simulink model "sampleModel1819"  (R2023a)
settings: Solver=VariableStepAuto  StartTime=0.0  StopTime=10.0  RelTol=1e-3
libraries: hdlsllib x4, simulink x2
settings Model: Creator=user1  LastModifiedBy=user1

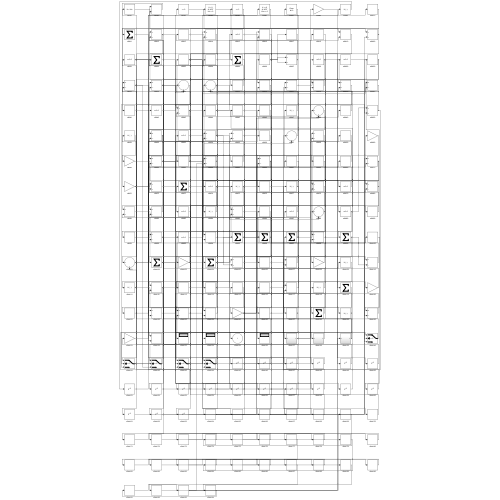
[thumbnail: Simulink's stored preview of the top-level diagram]
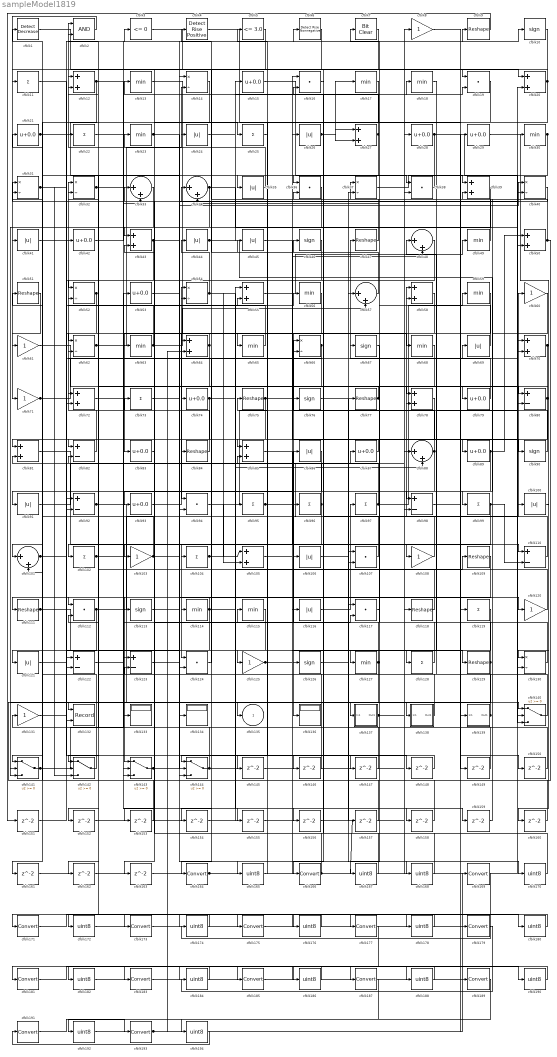
== system sampleModel1819 ==
  cfblk1 : simulink/Logic and Bit Operations/Detect Decrease  vinit=0.0  OutDataTypeStr=boolean
      settings: LibrarySourceBlock=|
      | hdlsllib/Logic and Bit
      | Operations/Detect
      | Decrease
  cfblk{10,46,67,76,90,113,126} (7 alike) : Signum
  cfblk{24,26,35,41,44..45,69,86,91,100,106,116,121} (13 alike) : Abs  SaturateOnIntegerOverflow=off
  cfblk{33..34,48,57,88,101} (6 alike) : Sum  Inputs=|++
  cfblk{11,22,25,73,95..97,99,102,104,119,128} (12 alike) : Sum  Inputs=+
  cfblk{8,60..61,71,103,108,120,125,131} (9 alike) : Gain
  cfblk{12,20,27,39,43,50,55,58,64,70,72,78,81,85,105} (15 alike) : Sum
  cfblk{16,19,36,38,94,107,112,117,124} (9 alike) : DotProduct  OutDataTypeStr=Inherit: Inherit via internal rule
  cfblk{9,47,51,75,77,84,109,111,118,129} (10 alike) : Reshape
  cfblk{80,82,92,98,110,122..123} (7 alike) : Sum  Inputs=+-
  cfblk{13,17..18,23,30,49,56,59,63,65,68,114..115,127} (14 alike) : MinMax
  cfblk{14,31..32,37,40,52,54,62,66,130} (10 alike) : Product  Inputs=*/  RndMeth=Zero  SaturateOnIntegerOverflow=on
  cfblk132 : Record  FileSettingsInternal="{\"entries\":[{\"content\":{\"excelSettings\":{\"content\":{},\"type\":\"Streamout.ExcelSettings\"}},\"type\":\"Streamout.FileSettingStorage\",\"uuid\":\"\"}],\"packageUris\":[\"http:\\/\\/schema.mathworks.com\\/mf0\\/streamout_blocks\\/R2020a\"],\"version\":\"1.0\"}"  Layout=[1 1]  SignalsInternal="{\"entries\":[{\"content\":{\"signals\":[{\"content\":{\"blockPath\":[],\"dimensions\":[1],\"domain\":\"\",\"lineColor\":\"#a2142f\",\"plots\":[1],\"port\":1,\"signalID\":4319,\"signalName\":\"XY Graph:1\"},\"type\":\"RecordBlkView.Signal\",\"uuid\":\"\"},{\"content\":{\"blockPath\":[],\"dimensions\":[1],\"domain\":\"\",\"lineColor\":\"#139fff\",\"plots\":[1],\"port\":2,\"signalID\":4322,\"signalName\":\"XY Graph:2\"},\"type\":\"RecordBlkView.Signal\",\"uuid\":\"\"}]},\"type\":\"RecordBlkView.InputSignals\",\"uuid\":\"\"}],\"packageUris\":[\"http:\\/\\/schema.mathworks.com\\/mf0\\/streamout_blocks\\/R2020a\"],\"version\":\"1.0\"}"  VisualizationBindings="{\"xyplotplugin\":{\"info\":[{\"series\":[{\"bindingParametersList\":[{\"parameter\":\"X-Axis\",\"signalID\":4319,\"signalName\":\"XY Graph:1\"},{\"parameter\":\"Y-Axis\",\"signalID\":4322,\"signalName\":\"XY Graph:2\"}],\"seriesID\":21637}],\"subplotID\":1}]}}"  CompatibilityTag=XY  st=-1
  cfblk133 : Display
  cfblk134 : Display
  cfblk136 : Display
  cfblk137 : Subsystem
      settings: LibrarySourceBlock=|
      | hdlsllib/Ports &
      | Subsystems/Subsystem
  cfblk138 : Subsystem
      settings: LibrarySourceBlock=|
      | hdlsllib/Ports &
      | Subsystems/Subsystem
  cfblk139 : Subsystem
      settings: LibrarySourceBlock=|
      | hdlsllib/Ports &
      | Subsystems/Subsystem
  cfblk{140..144} (5 alike) : Switch  SaturateOnIntegerOverflow=off  InputSameDT=off
  cfblk{145..163} (19 alike) : Delay  SampleTime=1
  cfblk{15,21,28..29,42,53,74,79,83,87,89,93} (12 alike) : Bias  Bias=0.0  SaturateOnIntegerOverflow=off
  cfblk{164,166,169,171,173,175,177,179,181,183,185,187,189,191,193} (15 alike) : DataTypeConversion  SaturateOnIntegerOverflow=off  RndMeth=Floor
  cfblk{165,167..168,170,172,174,176,178,180,182,184,186,188,190,192,194} (16 alike) : DataTypeConversion  OutDataTypeStr=uint8  SaturateOnIntegerOverflow=off  RndMeth=Floor
  cfblk2 : Logic  AllPortsSameDT=off  OutDataTypeStr=boolean
  cfblk3 : hdlsllib/Logic and Bit Operations/Compare To Zero  relop=<=  OutDataTypeStr=boolean
  cfblk4 : hdlsllib/Logic and Bit Operations/Detect Rise Positive  vinit=0  OutDataTypeStr=boolean
  cfblk5 : hdlsllib/Logic and Bit Operations/Compare To Constant  relop=<=  const=3.0  OutDataTypeStr=boolean
  cfblk6 : hdlsllib/Logic and Bit Operations/Detect Rise Nonnegative  vinit=0  OutDataTypeStr=boolean
  cfblk7 : simulink/Logic and Bit Operations/Bit Clear  iBit=0
      settings: LibrarySourceBlock=|
      | hdlsllib/Logic and Bit
      | Operations/Bit Clear
  cfblk135 : Outport  VectorParamsAs1DForOutWhenUnconnected=off
  wires:
  cfblk56/1 -> cfblk83/1
  cfblk13/1 -> cfblk65/1
  cfblk89/1 -> cfblk50/1, cfblk154/1
  cfblk1/1 -> cfblk20/1
  cfblk119/1 -> cfblk125/1
  cfblk54/1 -> cfblk44/1, cfblk105/2, cfblk156/1
  cfblk44/1 -> cfblk99/1, cfblk18/1
  cfblk95/1 -> cfblk60/1, cfblk80/2
  cfblk79/1 -> cfblk47/1
  cfblk49/1 -> cfblk23/1
  cfblk97/1 -> cfblk59/1, cfblk51/1
  cfblk144/1 -> cfblk131/1, cfblk98/2
  cfblk29/1 -> cfblk130/1
  cfblk108/1 -> cfblk58/1
  cfblk138/1(Out1) -> cfblk73/1
  cfblk59/1 -> cfblk136/1
  cfblk143/1 -> cfblk14/1, cfblk40/2
  cfblk96/1 -> cfblk102/1, cfblk82/2
  cfblk55/1 -> cfblk49/1
  cfblk93/1 -> cfblk54/1
  cfblk21/1 -> cfblk25/1, cfblk144/3, cfblk146/1
  cfblk92/1 -> cfblk137/1(In1), cfblk112/1
  cfblk130/1 -> cfblk86/1
  cfblk43/1 -> cfblk40/1, cfblk72/2
  cfblk50/1 -> cfblk132/1, cfblk24/1
  cfblk2/1 -> cfblk71/1
  cfblk19/1 -> cfblk98/1
  cfblk112/1 -> cfblk100/1, cfblk161/1
  cfblk128/1 -> cfblk7/1
  cfblk26/1 -> cfblk17/1, cfblk27/1, cfblk27/2
  cfblk127/1 -> cfblk33/1, cfblk163/1
  cfblk82/1 -> cfblk32/1
  cfblk23/1 -> cfblk134/1, cfblk76/1, cfblk96/1
  cfblk4/1 -> cfblk119/1
  cfblk7/1 -> cfblk106/1
  cfblk109/1 -> cfblk143/1
  cfblk91/1 -> cfblk87/1
  cfblk57/1 -> cfblk34/1
  cfblk10/1 -> cfblk41/1
  cfblk131/1 -> cfblk56/1
  cfblk14/1 -> cfblk123/1
  cfblk3/1 -> cfblk19/1
  cfblk20/1 -> cfblk35/1, cfblk11/1
  cfblk64/1 -> cfblk62/1, cfblk152/1
  cfblk38/1 -> cfblk36/1
  cfblk129/1 -> cfblk75/1, cfblk141/3
  cfblk99/1 -> cfblk124/1, cfblk110/2
  cfblk5/1 -> cfblk164/1
  cfblk103/1 -> cfblk31/1, cfblk165/1
  cfblk71/1 -> cfblk28/1, cfblk54/2
  cfblk126/1 -> cfblk77/1
  cfblk37/1 -> cfblk39/1
  cfblk62/1 -> cfblk14/2, cfblk94/2, cfblk148/1
  cfblk81/1 -> cfblk130/2
  cfblk61/1 -> cfblk79/1
  cfblk63/1 -> cfblk57/2, cfblk22/1, cfblk168/1
  cfblk116/1 -> cfblk97/1
  cfblk70/1 -> cfblk126/1, cfblk144/2
  cfblk90/1 -> cfblk48/1
  cfblk75/1 -> cfblk141/1, cfblk67/1
  cfblk40/1 -> cfblk31/2
  cfblk17/1 -> cfblk43/1
  cfblk125/1 -> cfblk48/2, cfblk129/1, cfblk78/2
  cfblk36/1 -> cfblk114/1
  cfblk30/1 -> cfblk128/1, cfblk133/1
  cfblk102/1 -> cfblk158/1, cfblk159/1
  cfblk80/1 -> cfblk93/1, cfblk78/1
  cfblk15/1 -> cfblk38/1
  cfblk85/1 -> cfblk107/2
  cfblk76/1 -> cfblk138/1(In1)
  cfblk69/1 -> cfblk34/2
  cfblk120/1 -> cfblk45/1
  cfblk72/1 -> cfblk55/2
  cfblk6/1 -> cfblk63/1
  cfblk33/1 -> cfblk141/2
  cfblk27/1 -> cfblk4/1, cfblk121/1
  cfblk46/1 -> cfblk122/2
  cfblk83/1 -> cfblk113/1
  cfblk68/1 -> cfblk94/1
  cfblk58/1 -> cfblk84/1
  cfblk51/1 -> cfblk61/1
  cfblk122/1 -> cfblk117/2
  cfblk18/1 -> cfblk108/1
  cfblk110/1 -> cfblk36/2
  cfblk113/1 -> cfblk66/1
  cfblk74/1 -> cfblk80/1, cfblk88/2, cfblk162/1
  cfblk52/1 -> cfblk132/2, cfblk92/2
  cfblk11/1 -> cfblk42/1
  cfblk124/1 -> cfblk64/1
  cfblk107/1 -> cfblk46/1
  cfblk35/1 -> cfblk2/1
  cfblk114/1 -> cfblk109/1, cfblk111/1, cfblk143/3
  cfblk39/1 -> cfblk101/1
  cfblk101/1 -> cfblk6/1, cfblk3/1
  cfblk31/1 -> cfblk124/2, cfblk142/3
  cfblk24/1 -> cfblk15/1
  cfblk104/1 -> cfblk105/1, cfblk69/1, cfblk95/1
  cfblk88/1 -> cfblk91/1, cfblk66/2
  cfblk22/1 -> cfblk68/1
  cfblk66/1 -> cfblk135/1, cfblk62/2
  cfblk65/1 -> cfblk12/1
  cfblk47/1 -> cfblk13/1
  cfblk12/1 -> cfblk81/1, cfblk155/1
  cfblk94/1 -> cfblk8/1
  cfblk140/1 -> cfblk123/2
  cfblk28/1 -> cfblk52/1, cfblk140/2
  cfblk77/1 -> cfblk74/1, cfblk127/1
  cfblk78/1 -> cfblk103/1
  cfblk73/1 -> cfblk120/1
  cfblk45/1 -> cfblk90/1
  cfblk118/1 -> cfblk72/1
  cfblk87/1 -> cfblk85/1
  cfblk105/1 -> cfblk110/1
  cfblk142/1 -> cfblk21/1
  cfblk111/1 -> cfblk81/2, cfblk143/2
  cfblk34/1 -> cfblk82/1, cfblk50/2
  cfblk141/1 -> cfblk53/1, cfblk142/2
  cfblk53/1 -> cfblk9/1
  cfblk16/1 -> cfblk166/1
  cfblk121/1 -> cfblk70/2
  cfblk32/1 -> cfblk142/1, cfblk140/3, cfblk33/2
  cfblk84/1 -> cfblk12/2
  cfblk41/1 -> cfblk140/1
  cfblk48/1 -> cfblk104/1
  cfblk117/1 -> cfblk37/1
  cfblk139/1(Out1) -> cfblk58/2, cfblk112/2
  cfblk60/1 -> cfblk89/1
  cfblk42/1 -> cfblk10/1
  cfblk137/1(Out1) -> cfblk88/1, cfblk19/2
  cfblk25/1 -> cfblk145/1
  cfblk145/1 -> cfblk57/1
  cfblk146/1 -> cfblk2/2
  cfblk123/1 -> cfblk147/1
  cfblk147/1 -> cfblk52/2
  cfblk148/1 -> cfblk144/1
  cfblk8/1 -> cfblk149/1
  cfblk149/1 -> cfblk101/2
  cfblk98/1 -> cfblk150/1
  cfblk150/1 -> cfblk32/2
  cfblk9/1 -> cfblk151/1
  cfblk151/1 -> cfblk122/1
  cfblk152/1 -> cfblk38/2
  cfblk86/1 -> cfblk153/1
  cfblk153/1 -> cfblk1/1
  cfblk154/1 -> cfblk55/1
  cfblk155/1 -> cfblk85/2
  cfblk156/1 -> cfblk37/2
  cfblk157/1 -> cfblk92/1
  cfblk158/1 -> cfblk107/1
  cfblk159/1 -> cfblk39/2
  cfblk100/1 -> cfblk160/1
  cfblk160/1 -> cfblk117/1
  cfblk161/1 -> cfblk20/2
  cfblk162/1 -> cfblk26/1
  cfblk163/1 -> cfblk70/1
  cfblk164/1 -> cfblk157/1, cfblk116/1
  cfblk165/1 -> cfblk5/1
  cfblk166/1 -> cfblk30/1, cfblk118/1, cfblk43/2
  cfblk67/1 -> cfblk167/1
  cfblk167/1 -> cfblk16/1
  cfblk168/1 -> cfblk16/2
  cfblk106/1 -> cfblk170/1
  cfblk170/1 -> cfblk115/1
  cfblk115/1 -> cfblk172/1
  cfblk172/1 -> cfblk169/1
  cfblk169/1 -> cfblk174/1
  cfblk174/1 -> cfblk171/1
  cfblk171/1 -> cfblk176/1
  cfblk176/1 -> cfblk173/1
  cfblk173/1 -> cfblk178/1
  cfblk178/1 -> cfblk175/1
  cfblk175/1 -> cfblk180/1
  cfblk180/1 -> cfblk177/1
  cfblk177/1 -> cfblk182/1
  cfblk182/1 -> cfblk179/1
  cfblk179/1 -> cfblk184/1
  cfblk184/1 -> cfblk181/1
  cfblk181/1 -> cfblk186/1
  cfblk186/1 -> cfblk183/1
  cfblk183/1 -> cfblk188/1
  cfblk188/1 -> cfblk185/1
  cfblk185/1 -> cfblk190/1
  cfblk190/1 -> cfblk187/1
  cfblk191/1 -> cfblk193/1
  cfblk187/1 -> cfblk192/1
  cfblk192/1 -> cfblk189/1
  cfblk193/1 -> cfblk29/1, cfblk139/1(In1), cfblk64/2
  cfblk189/1 -> cfblk194/1
  cfblk194/1 -> cfblk191/1

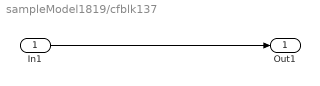
== system sampleModel1819/cfblk137 ==
  In1 : Inport
  Out1 : Outport
  wires:
  In1/1 -> Out1/1

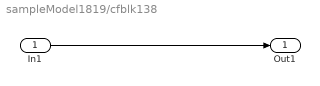
== system sampleModel1819/cfblk138 ==
  In1 : Inport
  Out1 : Outport
  wires:
  In1/1 -> Out1/1

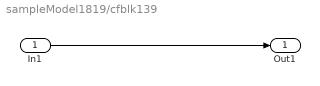
== system sampleModel1819/cfblk139 ==
  In1 : Inport
  Out1 : Outport
  wires:
  In1/1 -> Out1/1
